simulink model "foc_controlsystem_pwm"  (R2018a)
settings: Solver=ode23t  StartTime=0.0  StopTime=1  RelTol=1e-3
undefined symbols (not defined in the file): Dm, Ki_id, Ki_iq, Ki_s, Kp_id, Kp_iq, Kp_s, Ld, Lq, p, Phi, Ts, Vdc
libraries: nesl_utility x13, fl_lib x11, pe_lib x5, simulink x3, peTransforms x2, pePwmGeneratorTwoLevel x1, powerlib_meascontrol x1
Description:
  | % Copyright 2018 The MathWorks, Inc.
settings Model: SimulationMode=accelerator  Creator=kfukui  LastModifiedBy=kfukui
settings DataIOCC: SaveOutput=off  SignalLogging=off  DSMLogging=off  SaveTime=off

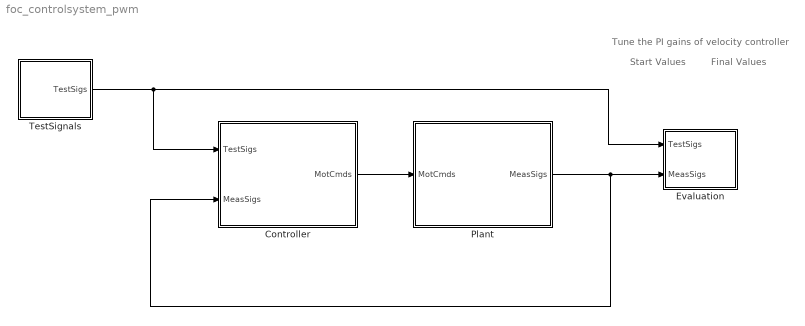
== system foc_controlsystem_pwm ==
  note: Tune the PI gains of velocity controller
  note: Start Values
  note: Final Values
  Controller : Subsystem
  Evaluation : Subsystem
  Plant : Subsystem
  TestSignals : Subsystem
  wires:
  Plant/1(MeasSigs) -> Evaluation/2(MeasSigs), Controller/2(MeasSigs)
  TestSignals/1(TestSigs) -> Evaluation/1(TestSigs), Controller/1(TestSigs)
  Controller/1(MotCmds) -> Plant/1(MotCmds)

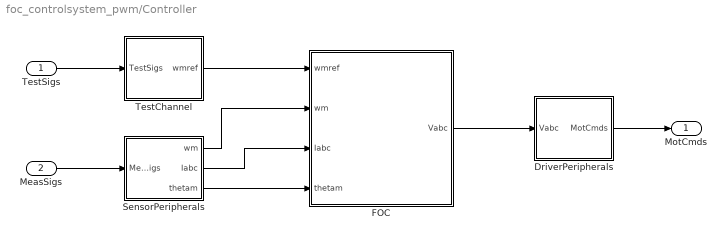
== system foc_controlsystem_pwm/Controller ==
  TestSigs : Inport
  MeasSigs : Inport  Port=2
  DriverPeripherals : Subsystem
  FOC : Subsystem
  SensorPeripherals : Subsystem
  TestChannel : Subsystem
  MotCmds : Outport
  wires:
  FOC/1(Vabc) -> DriverPeripherals/1(Vabc)
  DriverPeripherals/1(MotCmds) -> MotCmds/1
  TestSigs/1 -> TestChannel/1(TestSigs)
  TestChannel/1(wmref) -> FOC/1(wmref)
  MeasSigs/1 -> SensorPeripherals/1(MeasSigs)
  SensorPeripherals/1(wm) -> FOC/2(wm)
  SensorPeripherals/2(Iabc) -> FOC/3(Iabc)
  SensorPeripherals/3(thetam) -> FOC/4(thetam)

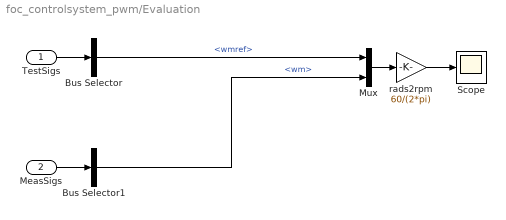
== system foc_controlsystem_pwm/Evaluation ==
  TestSigs : Inport
  MeasSigs : Inport  Port=2
  Bus Selector : BusSelector  OutputSignals=wmref
  Bus Selector1 : BusSelector  OutputSignals=wm
  Mux : Mux  Inputs=2
  Scope : Scope
  rads2rpm : Gain  Gain=60/(2*pi)
  wires:
  TestSigs/1 -> Bus Selector/1
  Mux/1 -> rads2rpm/1
  rads2rpm/1 -> Scope/1
  MeasSigs/1 -> Bus Selector1/1
  Bus Selector/1 -> Mux/1  "<wmref>"
  Bus Selector1/1 -> Mux/2  "<wm>"

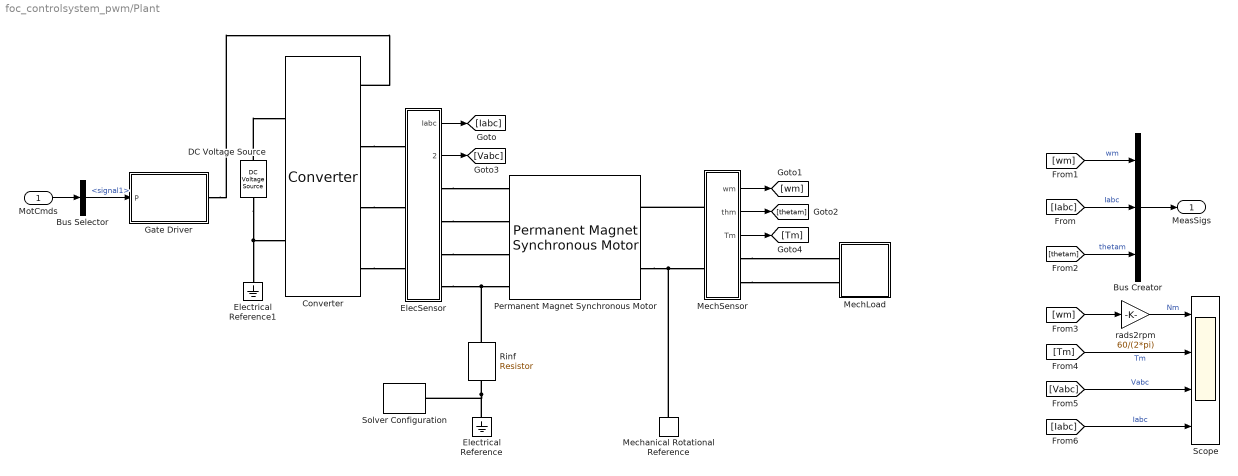
== system foc_controlsystem_pwm/Plant ==
  MotCmds : Inport
  Bus Creator : BusCreator  Inputs=3
  Bus Selector : BusSelector  OutputSignals=signal1
  Converter : pe_lib/Semiconductors/Converter  device_type=3  Vf=0.8 V  Ron=0.001 Ohm  Rds=0.001 Ohm  Goff=1e-6 1/Ohm  Vth=0.5 V  Vgt=1 V  Vgt_off=-1 V  Ih=1 A  diode_param=2  diode_Vf=0.8 V  diode_Ron=0.001 Ohm  diode_Goff=1e-5 1/Ohm  diode_C=50 nF  diode_iRM=-235 A  diode_iF=300 A  diode_idot=-50 A/us  diode_trr_param=1  diode_trr_factor=3  diode_trr=15 us  diode_Qrr=1.5e+3 s*uA  snubber_type=0  Rs=0.1 Ohm  Cs=1e-7 F
      settings: SourceProductName=Simscape Power Systems  SourceProductBaseCode=PS
  DC Voltage Source : fl_lib/Electrical/Electrical Sources/DC Voltage Source  v0=Vdc V
  ElecSensor : Subsystem
  Electrical Reference : fl_lib/Electrical/Electrical Elements/Electrical Reference
  Electrical Reference1 : fl_lib/Electrical/Electrical Elements/Electrical Reference
  Gate Driver : Subsystem
  MechLoad : Subsystem
  MechSensor : Subsystem
  Mechanical Rotational Reference : fl_lib/Mechanical/Rotational Elements/Mechanical Rotational Reference
  Permanent Magnet Synchronous Motor : pe_lib/Machines/Permanent Magnet Rotor/Permanent Magnet Synchronous Motor  nPolePairs=p  pmflux_param=1  pm_flux_linkage=Phi Wb  torque_constant=0.18 N*m/A  back_emf_constant=0.18 V/(rad/s)  stator_param=1  Ld=Ld H  Lq=Lq H  L0=0 H  Ls=0.0002 H  Lm=-0.00002 H  Ms=0.00002 H  Rs=Rs Ohm  zero_sequence=pe.enum.park.zerosequence.exclude  J=0 kg*m^2  lam=0 N*m/(rad/s)  axes_param=2  i_d_specify=off  i_d_priority=None  i_d=0 A  i_d_nominal_specify=off  i_d_nominal_unit=A  i_d_nominal_value=1  i_q_specify=off  i_q_priority=None  i_q=0 A  i_q_nominal_specify=off  i_q_nominal_unit=A  i_q_nominal_value=1  torque_specify=off  torque_priority=None  torque=0 N*m  torque_nominal_specify=off  torque_nominal_unit=N*m  torque_nominal_value=1  angular_velocity_specify=off  angular_velocity_priority=High  angular_velocity=0 rpm  angular_velocity_nominal_specify=off  angular_velocity_nominal_unit=rpm  angular_velocity_nominal_value=1  angular_position_specify=off  angular_position_priority=High  angular_position=0 deg  angular_position_nominal_specify=off  angular_position_nominal_unit=deg  angular_position_nominal_value=1
      settings: SourceProductName=Simscape Power Systems  SourceProductBaseCode=PS
  Rinf : fl_lib/Electrical/Electrical Elements/Resistor  R=1e9 Ohm  i_specify=off  i_priority=None  i=0 A  i_nominal_specify=off  i_nominal_unit=A  i_nominal_value=1  v_specify=off  v_priority=None  v=0 V  v_nominal_specify=off  v_nominal_unit=V  v_nominal_value=1
  Scope : Scope  NumInputPorts=4
  Solver Configuration : nesl_utility/Solver Configuration  PhysicalDomain=network_engine_domain  SubClassName=solver  LeftPortType=input  RightPortType=generic  Tones=[]  Harmonics=[]  SimulateNoise=off  Profile=off  UseLocalSampling=off  EnableSwitchedLinearOptims=on  FrequencyDomain=off  UseCCode=off  RelTol=0.001  AbsTol=1e-06  MinStep=1e-09  ToWorkspace=off  RevertToSquareIcSolve=off  NumHomotopyIterations=100  PhasorMode=off  PhasorModeNumHarmonics=1  DoDC=off  ResidualTolerance=1e-09  UseLocalSolver=on  LocalSolverChoice=NE_PARTITIONING_ADVANCER  LocalSolverSampleTime=Ts  DoFixedCost=on  MaxNonlinIter=4  MaxModeIter=2  LinearAlgebra=Sparse  EquationFormulation=NE_TIME_EF  DelaysMemoryBudget=1024  AutomaticFiltering=on  FilteringTimeConstant=0.001
  rads2rpm : Gain  Gain=60/(2*pi)
  MeasSigs : Outport
  wires:
  ElecSensor/1(Iabc) -> [Iabc]
  ElecSensor/2(Vabc) -> [Vabc]
  MechSensor/1(wm) -> [wm]
  MechSensor/2(thm) -> [thetam]
  MechSensor/3(Tm) -> [Tm]
  [wm] -> Bus Creator/1  "wm"
  [Iabc] -> Bus Creator/2  "Iabc"
  [thetam] -> Bus Creator/3  "thetam"
  Bus Creator/1 -> MeasSigs/1
  MotCmds/1 -> Bus Selector/1
  Bus Selector/1 -> Gate Driver/1(P)  "<signal1>"
  rads2rpm/1 -> Scope/1  "Nm"
  [Tm] -> Scope/2  "Tm"
  [Vabc] -> Scope/3  "Vabc"
  [Iabc] -> Scope/4  "Iabc"
  [wm] -> rads2rpm/1
  connections:
  ElecSensor/RConn3 -- Permanent Magnet Synchronous Motor/LConn3
  Rinf/LConn1 -- ElecSensor/RConn4 -- Permanent Magnet Synchronous Motor/LConn4
  Converter/LConn3 -- ElecSensor/LConn2
  Rinf/RConn1 -- Electrical Reference/LConn1 -- Solver Configuration/RConn1
  ElecSensor/RConn2 -- Permanent Magnet Synchronous Motor/LConn2
  ElecSensor/RConn1 -- Permanent Magnet Synchronous Motor/LConn1
  Converter/LConn4 -- ElecSensor/LConn3
  Converter/LConn2 -- ElecSensor/LConn1
  Permanent Magnet Synchronous Motor/RConn2 -- Mechanical Rotational Reference/LConn1 -- MechSensor/LConn2
  MechSensor/RConn1 -- MechLoad/LConn1
  MechSensor/LConn1 -- Permanent Magnet Synchronous Motor/RConn1
  Gate Driver/RConn1 -- Converter/LConn1
  DC Voltage Source/LConn1 -- Converter/RConn1
  DC Voltage Source/RConn1 -- Electrical Reference1/LConn1 -- Converter/RConn2
  MechSensor/RConn2 -- MechLoad/LConn2

== system foc_controlsystem_pwm/TestSignals ==
  Bus Creator : BusCreator  Inputs=1
  Nmref : Step  Time=0.05  After=1000  SampleTime=0
  rpm2rads : Gain  Gain=2*pi/60
  TestSigs : Outport
  wires:
  Nmref/1 -> rpm2rads/1
  rpm2rads/1 -> Bus Creator/1  "wmref"
  Bus Creator/1 -> TestSigs/1

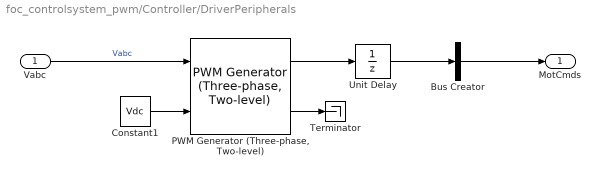
== system foc_controlsystem_pwm/Controller/DriverPeripherals ==
  Vabc : Inport
  Bus Creator : BusCreator  Inputs=1
  Constant1 : Constant  Value=Vdc
  "PWM Generator (Three-phase, Two-level)" : pePwmGeneratorTwoLevel/PWM Generator (Three-phase, Two-level)  OverrideUsingVariant=NaturalMode  PWMMode=Continuous PWM (CPWM)  CPWMMode=SPWM: sinusoidal PWM  DPWMMode=60 DPWM: 60 degree discontinuous PWM  fsw=fc  Ts=Ts
      settings: SamplingMode=Natural
  Terminator : Terminator
  Unit Delay : UnitDelay  SampleTime=-1
  MotCmds : Outport
  wires:
  Bus Creator/1 -> MotCmds/1
  Constant1/1 -> "PWM Generator (Three-phase, Two-level)"/2
  Vabc/1 -> "PWM Generator (Three-phase, Two-level)"/1  "Vabc"
  "PWM Generator (Three-phase, Two-level)"/1 -> Unit Delay/1
  "PWM Generator (Three-phase, Two-level)"/2 -> Terminator/1
  Unit Delay/1 -> Bus Creator/1

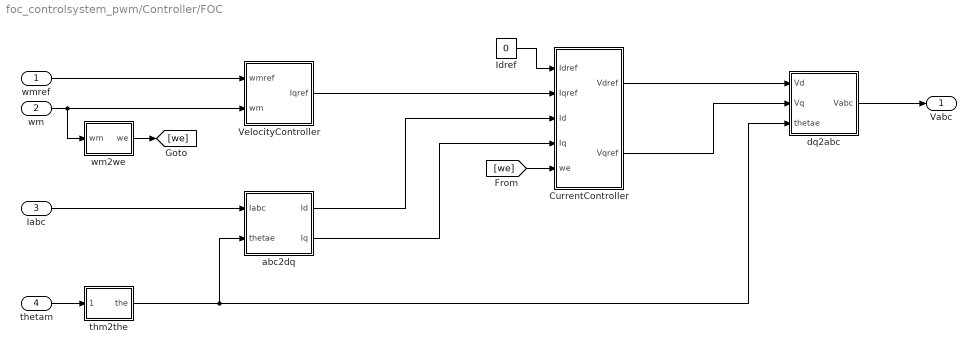
== system foc_controlsystem_pwm/Controller/FOC ==
  wmref : Inport
  wm : Inport  Port=2
  Iabc : Inport  Port=3
  thetam : Inport  Port=4
  CurrentController : Subsystem
  Idref : Constant  Value=0  SampleTime=-1
  VelocityController : Subsystem
  abc2dq : Subsystem
  dq2abc : Subsystem
  thm2the : Subsystem
  wm2we : Subsystem
  Vabc : Outport
  wires:
  abc2dq/2(Iq) -> CurrentController/4(Iq)
  wmref/1 -> VelocityController/1(wmref)
  abc2dq/1(Id) -> CurrentController/3(Id)
  Iabc/1 -> abc2dq/1(Iabc)
  CurrentController/1(Vdref) -> dq2abc/1(Vd)
  CurrentController/2(Vqref) -> dq2abc/2(Vq)
  [we] -> CurrentController/5(we)
  wm/1 -> VelocityController/2(wm), wm2we/1(wm)
  Idref/1 -> CurrentController/1(Idref)
  dq2abc/1(Vabc) -> Vabc/1
  VelocityController/1(Iqref) -> CurrentController/2(Iqref)
  thm2the/1(the) -> abc2dq/2(thetae), dq2abc/3(thetae)
  thetam/1 -> thm2the/1(thm)
  wm2we/1(we) -> [we]

== system foc_controlsystem_pwm/Controller/SensorPeripherals ==
  MeasSigs : Inport
  Bus Selector : BusSelector  OutputSignals=wm,Iabc,thetam
  wm : Outport
  Iabc : Outport  Port=2
  thetam : Outport  Port=3
  wires:
  MeasSigs/1 -> Bus Selector/1
  Bus Selector/2 -> Iabc/1  "<Iabc>"
  Bus Selector/1 -> wm/1  "<wm>"
  Bus Selector/3 -> thetam/1  "<thetam>"

== system foc_controlsystem_pwm/Controller/TestChannel ==
  TestSigs : Inport
  Bus Selector : BusSelector  OutputSignals=wmref
  wmref : Outport
  wires:
  TestSigs/1 -> Bus Selector/1
  Bus Selector/1 -> wmref/1  "<wmref>"

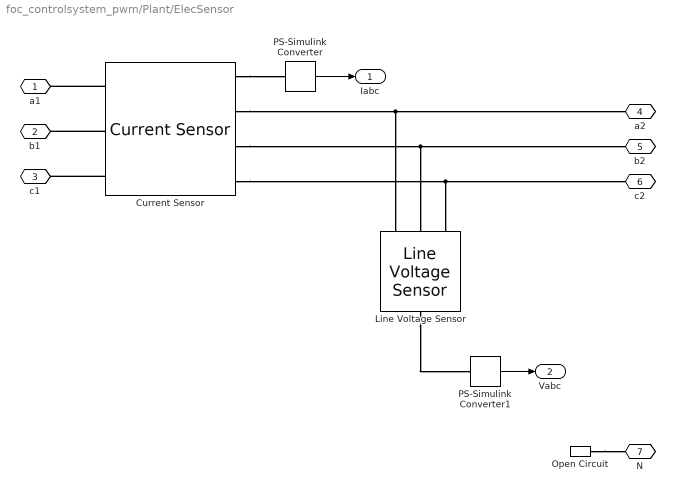
== system foc_controlsystem_pwm/Plant/ElecSensor ==
  Current Sensor : pe_lib/Sensors/Current Sensor
      settings: SourceProductName=Simscape Power Systems  SourceProductBaseCode=PS
  Line Voltage Sensor : pe_lib/Sensors/Line Voltage Sensor
      settings: SourceProductName=Simscape Power Systems  SourceProductBaseCode=PS
  Open Circuit : fl_lib/Electrical/Electrical Elements/Open Circuit  v_specify=off  v_priority=None  v=0 V  v_nominal_specify=off  v_nominal_unit=V  v_nominal_value=1
      settings: SourceProductName=Simscape  SourceProductBaseCode=SS
  PS-Simulink Converter : nesl_utility/PS-Simulink Converter  PhysicalDomain=network_engine_domain  SubClassName=ps_output  LeftPortType=input  RightPortType=output  PseudoPeriodic=off  Frequencies=[]  Unit=1  AffineConversion=off
  PS-Simulink Converter1 : nesl_utility/PS-Simulink Converter  PhysicalDomain=network_engine_domain  SubClassName=ps_output  LeftPortType=input  RightPortType=output  PseudoPeriodic=off  Frequencies=[]  Unit=1  AffineConversion=off
  a1 : PMIOPort  Side=Left
  b1 : PMIOPort  Port=2  Side=Left
  c1 : PMIOPort  Port=3  Side=Left
  a2 : PMIOPort  Port=4  Side=Right
  b2 : PMIOPort  Port=5  Side=Right
  c2 : PMIOPort  Port=6  Side=Right
  N : PMIOPort  Port=7  Side=Right
  Iabc : Outport
  Vabc : Outport  Port=2
  wires:
  PS-Simulink Converter/1 -> Iabc/1
  PS-Simulink Converter1/1 -> Vabc/1
  connections:
  Current Sensor/LConn1 -- a1/RConn1
  Current Sensor/LConn2 -- b1/RConn1
  Current Sensor/LConn3 -- c1/RConn1
  Current Sensor/RConn1 -- PS-Simulink Converter/LConn1
  Open Circuit/LConn1 -- N/RConn1
  Current Sensor/RConn2 -- Line Voltage Sensor/LConn1 -- a2/RConn1
  Current Sensor/RConn3 -- Line Voltage Sensor/LConn2 -- b2/RConn1
  Current Sensor/RConn4 -- Line Voltage Sensor/LConn3 -- c2/RConn1
  Line Voltage Sensor/RConn1 -- PS-Simulink Converter1/LConn1

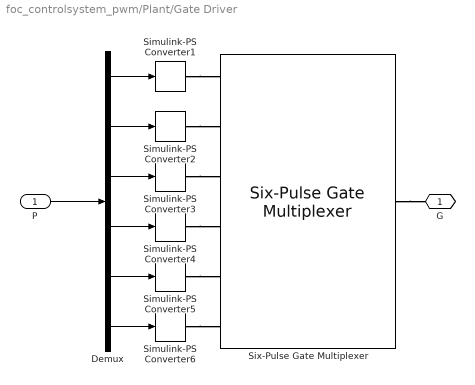
== system foc_controlsystem_pwm/Plant/Gate Driver ==
  P : Inport
  Demux : Demux  Outputs=6
  Simulink-PS Converter{1..6} (6 alike) : nesl_utility/Simulink-PS Converter  PhysicalDomain=network_engine_domain  SubClassName=ps_input  LeftPortType=input  RightPortType=output  PseudoPeriodic=off  Frequencies=[]  NoiseDistribution=none  NoiseParameters=[]  Unit=1  AffineConversion=off  FilteringAndDerivatives=provide  SimscapeFilterOrder=1  InputFilterTimeConstant=0.001  UdotUserProvided=0
  Six-Pulse Gate Multiplexer : pe_lib/Semiconductors/Six-Pulse Gate Multiplexer  R=0 Ohm
      settings: SourceProductName=Simscape Power Systems  SourceProductBaseCode=PS
  G : PMIOPort  Side=Right
  wires:
  Demux/6 -> Simulink-PS Converter6/1
  Demux/3 -> Simulink-PS Converter3/1
  Demux/4 -> Simulink-PS Converter4/1
  Demux/2 -> Simulink-PS Converter2/1
  Demux/5 -> Simulink-PS Converter5/1
  Demux/1 -> Simulink-PS Converter1/1
  P/1 -> Demux/1
  connections:
  Simulink-PS Converter1/RConn1 -- Six-Pulse Gate Multiplexer/LConn1
  Simulink-PS Converter5/RConn1 -- Six-Pulse Gate Multiplexer/LConn5
  Simulink-PS Converter3/RConn1 -- Six-Pulse Gate Multiplexer/LConn3
  Simulink-PS Converter4/RConn1 -- Six-Pulse Gate Multiplexer/LConn4
  Simulink-PS Converter2/RConn1 -- Six-Pulse Gate Multiplexer/LConn2
  Six-Pulse Gate Multiplexer/RConn1 -- G/RConn1
  Simulink-PS Converter6/RConn1 -- Six-Pulse Gate Multiplexer/LConn6

== system foc_controlsystem_pwm/Plant/MechLoad ==
  Ideal Torque Source : fl_lib/Mechanical/Mechanical Sources/Ideal Torque Source
  Inertia : fl_lib/Mechanical/Rotational Elements/Inertia  inertia=Jm kg*m^2  w_specify=off  w_priority=High  w=0 rad/s  w_nominal_specify=off  w_nominal_unit=rad/s  w_nominal_value=1  t_specify=off  t_priority=None  t=0 N*m  t_nominal_specify=off  t_nominal_unit=N*m  t_nominal_value=1
  Rotational Damper : fl_lib/Mechanical/Rotational Elements/Rotational Damper  D=Dm N*m/(rad/s)  w_specify=off  w_priority=None  w=0 rad/s  w_nominal_specify=off  w_nominal_unit=rad/s  w_nominal_value=1  t_specify=off  t_priority=None  t=0 N*m  t_nominal_specify=off  t_nominal_unit=N*m  t_nominal_value=1
  Simulink-PS Converter4 : nesl_utility/Simulink-PS Converter  PhysicalDomain=network_engine_domain  SubClassName=ps_input  LeftPortType=input  RightPortType=output  PseudoPeriodic=off  Frequencies=[]  NoiseDistribution=none  NoiseParameters=[]  Unit=1  AffineConversion=off  FilteringAndDerivatives=provide  SimscapeFilterOrder=1  InputFilterTimeConstant=0.001  UdotUserProvided=0
  Step : Step  Time=0.5  After=-0.2  SampleTime=0
  R : PMIOPort  Side=Left
  C : PMIOPort  Port=2  Side=Left
  wires:
  Step/1 -> Simulink-PS Converter4/1
  connections:
  Ideal Torque Source/RConn1 -- Simulink-PS Converter4/RConn1
  Ideal Torque Source/RConn2 -- Rotational Damper/RConn1 -- C/RConn1
  Ideal Torque Source/LConn1 -- Rotational Damper/LConn1 -- R/RConn1 -- Inertia/LConn1

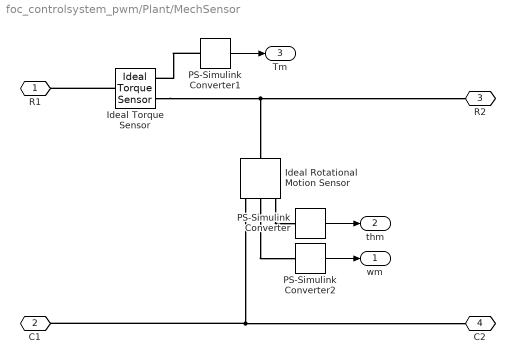
== system foc_controlsystem_pwm/Plant/MechSensor ==
  Ideal Rotational Motion Sensor : fl_lib/Mechanical/Mechanical Sensors/Ideal Rotational Motion Sensor  offset=0 rad
  Ideal Torque Sensor : fl_lib/Mechanical/Mechanical Sensors/Ideal Torque Sensor
  PS-Simulink Converter : nesl_utility/PS-Simulink Converter  PhysicalDomain=network_engine_domain  SubClassName=ps_output  LeftPortType=input  RightPortType=output  PseudoPeriodic=off  Frequencies=[]  Unit=1  AffineConversion=off
  PS-Simulink Converter1 : nesl_utility/PS-Simulink Converter  PhysicalDomain=network_engine_domain  SubClassName=ps_output  LeftPortType=input  RightPortType=output  PseudoPeriodic=off  Frequencies=[]  Unit=1  AffineConversion=off
  PS-Simulink Converter2 : nesl_utility/PS-Simulink Converter  PhysicalDomain=network_engine_domain  SubClassName=ps_output  LeftPortType=input  RightPortType=output  PseudoPeriodic=off  Frequencies=[]  Unit=1  AffineConversion=off
  R1 : PMIOPort  Side=Left
  C1 : PMIOPort  Port=2  Side=Left
  R2 : PMIOPort  Port=3  Side=Right
  C2 : PMIOPort  Port=4  Side=Right
  wm : Outport
  thm : Outport  Port=2
  Tm : Outport  Port=3
  wires:
  PS-Simulink Converter/1 -> thm/1
  PS-Simulink Converter1/1 -> Tm/1
  PS-Simulink Converter2/1 -> wm/1
  connections:
  Ideal Rotational Motion Sensor/RConn3 -- PS-Simulink Converter/LConn1
  Ideal Rotational Motion Sensor/RConn1 -- C2/RConn1 -- C1/RConn1
  Ideal Torque Sensor/LConn1 -- R1/RConn1
  Ideal Torque Sensor/RConn1 -- R2/RConn1 -- Ideal Rotational Motion Sensor/LConn1
  PS-Simulink Converter1/LConn1 -- Ideal Torque Sensor/RConn2
  Ideal Rotational Motion Sensor/RConn2 -- PS-Simulink Converter2/LConn1

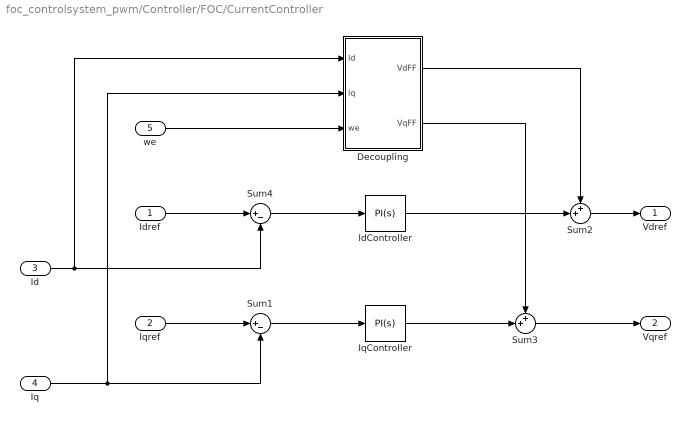
== system foc_controlsystem_pwm/Controller/FOC/CurrentController ==
  Idref : Inport
  Iqref : Inport  Port=2
  Id : Inport  Port=3
  Iq : Inport  Port=4
  we : Inport  Port=5
  Decoupling : Subsystem
  IdController : simulink/Continuous/PID Controller  Controller=PI  TimeDomain=Continuous-time  SampleTime=-1  IntegratorMethod=Forward Euler  FilterMethod=Forward Euler  Form=Parallel  UseFilter=on  ControllerParametersSource=internal  P=Kp_id  I=Ki_id  D=0  N=100  InitialConditionSource=internal  InitialConditionForIntegrator=0  InitialConditionForFilter=0  ExternalReset=none  LimitOutput=off  UpperSaturationLimit=inf  LowerSaturationLimit=-inf  LinearizeAsGain=on  AntiWindupMode=none  Kb=1  TrackingMode=off  Kt=1  PParamMin=[]  PParamMax=[]  IParamMin=[]  IParamMax=[]  DParamMin=[]  DParamMax=[]  NParamMin=[]  NParamMax=[]  KbParamMin=[]  KbParamMax=[]  KtParamMin=[]  KtParamMax=[]  POutMin=[]  POutMax=[]  IOutMin=[]  IOutMax=[]  DOutMin=[]  DOutMax=[]  NOutMin=[]  NOutMax=[]  KbOutMin=[]  KbOutMax=[]  KtOutMin=[]  KtOutMax=[]  IntegratorOutMin=[]  IntegratorOutMax=[]  FilterOutMin=[]  FilterOutMax=[]  SumOutMin=[]  SumOutMax=[]  SumI1OutMin=[]  SumI1OutMax=[]  SumI2OutMin=[]  SumI2OutMax=[]  SumI3OutMin=[]  SumI3OutMax=[]  SumDOutMin=[]  SumDOutMax=[]  SaturationOutMin=[]  SaturationOutMax=[]  IntegratorContinuousStateAttributes=''  IntegratorStateMustResolveToSignalObject=off  IntegratorRTWStateStorageClass=Auto  FilterContinuousStateAttributes=''  FilterStateMustResolveToSignalObject=off  FilterRTWStateStorageClass=Auto  DifferentiatorICPrevScaledInput=0  DifferentiatorOutMin=[]  DifferentiatorOutMax=[]  FilterDiffOutCoefMin=[]  FilterDiffOutCoefMax=[]  SumDenOutMin=[]  SumDenOutMax=[]  SumNumOutMin=[]  SumNumOutMax=[]  ReciprocalOutMin=[]  ReciprocalOutMax=[]  DivideOutMin=[]  DivideOutMax=[]  TunerSelectOption=Transfer Function Based (PID Tuner App)
  IqController : simulink/Continuous/PID Controller  Controller=PI  TimeDomain=Continuous-time  SampleTime=-1  IntegratorMethod=Forward Euler  FilterMethod=Forward Euler  Form=Parallel  UseFilter=on  ControllerParametersSource=internal  P=Kp_iq  I=Ki_iq  D=0  N=100  InitialConditionSource=internal  InitialConditionForIntegrator=0  InitialConditionForFilter=0  ExternalReset=none  LimitOutput=off  UpperSaturationLimit=inf  LowerSaturationLimit=-inf  LinearizeAsGain=on  AntiWindupMode=none  Kb=1  TrackingMode=off  Kt=1  PParamMin=[]  PParamMax=[]  IParamMin=[]  IParamMax=[]  DParamMin=[]  DParamMax=[]  NParamMin=[]  NParamMax=[]  KbParamMin=[]  KbParamMax=[]  KtParamMin=[]  KtParamMax=[]  POutMin=[]  POutMax=[]  IOutMin=[]  IOutMax=[]  DOutMin=[]  DOutMax=[]  NOutMin=[]  NOutMax=[]  KbOutMin=[]  KbOutMax=[]  KtOutMin=[]  KtOutMax=[]  IntegratorOutMin=[]  IntegratorOutMax=[]  FilterOutMin=[]  FilterOutMax=[]  SumOutMin=[]  SumOutMax=[]  SumI1OutMin=[]  SumI1OutMax=[]  SumI2OutMin=[]  SumI2OutMax=[]  SumI3OutMin=[]  SumI3OutMax=[]  SumDOutMin=[]  SumDOutMax=[]  SaturationOutMin=[]  SaturationOutMax=[]  IntegratorContinuousStateAttributes=''  IntegratorStateMustResolveToSignalObject=off  IntegratorRTWStateStorageClass=Auto  FilterContinuousStateAttributes=''  FilterStateMustResolveToSignalObject=off  FilterRTWStateStorageClass=Auto  DifferentiatorICPrevScaledInput=0  DifferentiatorOutMin=[]  DifferentiatorOutMax=[]  FilterDiffOutCoefMin=[]  FilterDiffOutCoefMax=[]  SumDenOutMin=[]  SumDenOutMax=[]  SumNumOutMin=[]  SumNumOutMax=[]  ReciprocalOutMin=[]  ReciprocalOutMax=[]  DivideOutMin=[]  DivideOutMax=[]  TunerSelectOption=Transfer Function Based (PID Tuner App)
  Sum1 : Sum  Inputs=|+-
  Sum2 : Sum  Inputs=++|
  Sum3 : Sum  Inputs=++|
  Sum4 : Sum  Inputs=|+-
  Vdref : Outport
  Vqref : Outport  Port=2
  wires:
  we/1 -> Decoupling/3(we)
  Idref/1 -> Sum4/1
  Sum2/1 -> Vdref/1
  Sum3/1 -> Vqref/1
  Iqref/1 -> Sum1/1
  Iq/1 -> Decoupling/2(Iq), Sum1/2
  Id/1 -> Decoupling/1(Id), Sum4/2
  Sum4/1 -> IdController/1
  Sum1/1 -> IqController/1
  Decoupling/2(VqFF) -> Sum3/1
  Decoupling/1(VdFF) -> Sum2/1
  IdController/1 -> Sum2/2
  IqController/1 -> Sum3/2

== system foc_controlsystem_pwm/Controller/FOC/VelocityController ==
  wmref : Inport
  wm : Inport  Port=2
  Gain : Gain  Gain=1/(3/2*p*Phi)
  PIDController : simulink/Continuous/PID Controller  Controller=PI  TimeDomain=Continuous-time  SampleTime=-1  IntegratorMethod=Forward Euler  FilterMethod=Forward Euler  Form=Parallel  UseFilter=on  ControllerParametersSource=internal  P=Kp_s  I=Ki_s  D=0  N=100  InitialConditionSource=internal  InitialConditionForIntegrator=0  InitialConditionForFilter=0  ExternalReset=none  LimitOutput=off  UpperSaturationLimit=inf  LowerSaturationLimit=-inf  LinearizeAsGain=on  AntiWindupMode=none  Kb=1  TrackingMode=off  Kt=1  PParamMin=[]  PParamMax=[]  IParamMin=[]  IParamMax=[]  DParamMin=[]  DParamMax=[]  NParamMin=[]  NParamMax=[]  KbParamMin=[]  KbParamMax=[]  KtParamMin=[]  KtParamMax=[]  POutMin=[]  POutMax=[]  IOutMin=[]  IOutMax=[]  DOutMin=[]  DOutMax=[]  NOutMin=[]  NOutMax=[]  KbOutMin=[]  KbOutMax=[]  KtOutMin=[]  KtOutMax=[]  IntegratorOutMin=[]  IntegratorOutMax=[]  FilterOutMin=[]  FilterOutMax=[]  SumOutMin=[]  SumOutMax=[]  SumI1OutMin=[]  SumI1OutMax=[]  SumI2OutMin=[]  SumI2OutMax=[]  SumI3OutMin=[]  SumI3OutMax=[]  SumDOutMin=[]  SumDOutMax=[]  SaturationOutMin=[]  SaturationOutMax=[]  IntegratorContinuousStateAttributes=''  IntegratorStateMustResolveToSignalObject=off  IntegratorRTWStateStorageClass=Auto  FilterContinuousStateAttributes=''  FilterStateMustResolveToSignalObject=off  FilterRTWStateStorageClass=Auto  DifferentiatorICPrevScaledInput=0  DifferentiatorOutMin=[]  DifferentiatorOutMax=[]  FilterDiffOutCoefMin=[]  FilterDiffOutCoefMax=[]  SumDenOutMin=[]  SumDenOutMax=[]  SumNumOutMin=[]  SumNumOutMax=[]  ReciprocalOutMin=[]  ReciprocalOutMax=[]  DivideOutMin=[]  DivideOutMax=[]  TunerSelectOption=Transfer Function Based (PID Tuner App)
  Sum : Sum  Inputs=|+-
  Iqref : Outport
  wires:
  PIDController/1 -> Gain/1
  Gain/1 -> Iqref/1
  wmref/1 -> Sum/1
  Sum/1 -> PIDController/1
  wm/1 -> Sum/2

== system foc_controlsystem_pwm/Controller/FOC/abc2dq ==
  Iabc : Inport
  thetae : Inport  Port=2
  Demux1 : Demux  Outputs=3
  Park Transform : peTransforms/Park Transform  AxisAlignment=D-axis  PowerInvariant=off
  Terminator : Terminator
  Id : Outport
  Iq : Outport  Port=2
  wires:
  Iabc/1 -> Park Transform/1
  thetae/1 -> Park Transform/2
  Demux1/3 -> Terminator/1
  Park Transform/1 -> Demux1/1
  Demux1/1 -> Id/1
  Demux1/2 -> Iq/1

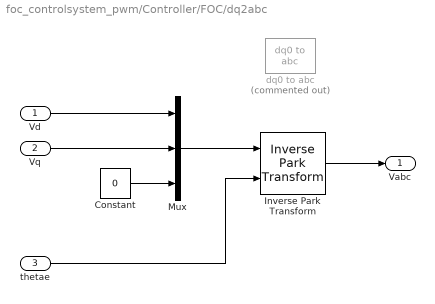
== system foc_controlsystem_pwm/Controller/FOC/dq2abc ==
  Vd : Inport
  Vq : Inport  Port=2
  thetae : Inport  Port=3
  Constant : Constant  Value=0
  Inverse Park Transform : peTransforms/Inverse Park Transform  AxisAlignment=D-axis  PowerInvariant=off
  Mux : Mux  Inputs=3
  dq0 to abc : powerlib_meascontrol/Transformations/dq0 to abc  Commented=on  Alignment=Aligned with phase A axis
  Vabc : Outport
  wires:
  thetae/1 -> Inverse Park Transform/2
  Constant/1 -> Mux/3
  Mux/1 -> Inverse Park Transform/1
  Vd/1 -> Mux/1
  Inverse Park Transform/1 -> Vabc/1
  Vq/1 -> Mux/2

== system foc_controlsystem_pwm/Controller/FOC/thm2the ==
  thm : Inport
  Constant : Constant  Value=2*pi
  Mod : Math  Operator=mod  SaturateOnIntegerOverflow=on
  PolePairs : Gain  Gain=p
  the : Outport
  wires:
  Constant/1 -> Mod/2
  PolePairs/1 -> Mod/1
  Mod/1 -> the/1
  thm/1 -> PolePairs/1

== system foc_controlsystem_pwm/Controller/FOC/wm2we ==
  wm : Inport
  PolePairs : Gain  Gain=p
  we : Outport
  wires:
  wm/1 -> PolePairs/1
  PolePairs/1 -> we/1

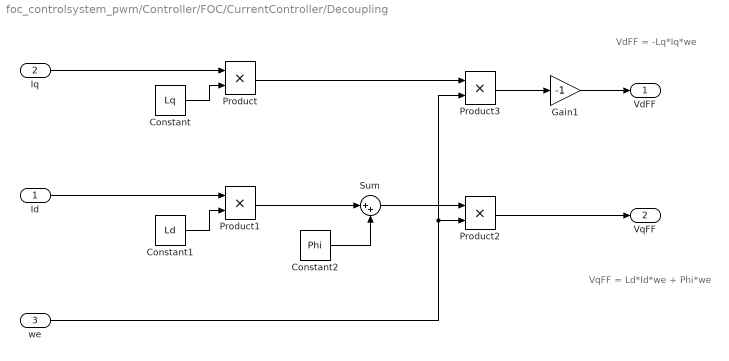
== system foc_controlsystem_pwm/Controller/FOC/CurrentController/Decoupling ==
  note: VdFF = -Lq*Iq*we
  note: VqFF = Ld*Id*we + Phi*we
  Id : Inport
  Iq : Inport  Port=2
  we : Inport  Port=3
  Constant : Constant  Value=Lq
  Constant1 : Constant  Value=Ld
  Constant2 : Constant  Value=Phi
  Gain1 : Gain  Gain=-1
  Product{,1..3} (4 alike) : Product
  Sum : Sum  Inputs=|++
  VdFF : Outport
  VqFF : Outport  Port=2
  wires:
  we/1 -> Product3/2, Product2/2
  Product1/1 -> Sum/1
  Constant2/1 -> Sum/2
  Sum/1 -> Product2/1
  Constant1/1 -> Product1/2
  Id/1 -> Product1/1
  Iq/1 -> Product/1
  Constant/1 -> Product/2
  Product3/1 -> Gain1/1
  Product/1 -> Product3/1
  Gain1/1 -> VdFF/1
  Product2/1 -> VqFF/1
